simulink model "component_contoller_PID"  (R2025a)
settings: Solver=FixedStepAuto  StartTime=0.0  StopTime=10.0  RelTol=1e-3  EnableMultiTasking=on
undefined symbols (not defined in the file): break_pedal_percentage, gas_pedal_percentage, steering_wheel_angle
libraries: slpidlib x1, drivingvehiclecontroller x1
settings Model: Creator=chmurski  LastModifiedBy=MarikL
settings SolverCC: AlgebraicLoopSolver=TrustRegion  PositivePriorityOrder=on
settings OptimizationCC: EnhancedBackFolding=on  PassReuseOutputArgsAs=Individual arguments  ZeroExternalMemoryAtStartup=off  ZeroInternalMemoryAtStartup=off  MaxStackSize=2048  OptimizeBlockOrder=speed  DifferentSizesBufferReuse=on  OptimizationCustomize=off  EfficientTunableParamExpr=on
settings DebuggingCC: ParameterTunabilityLossMsg=error  UnconnectedInputMsg=warning  UnconnectedOutputMsg=warning  UnconnectedLineMsg=warning
settings HardwareCC: ProdBitPerPointer=32.0  ProdBitPerSizeT=32.0  ProdBitPerPtrDiffT=32.0  ProdLargestAtomicInteger=Long  ProdWordSize=32.0  ProdLongLongMode=on  ProdHWDeviceType=Infineon->TriCore
settings ModelReferenceCC: EnableRefExpFcnMdlSchedulingChecks=on  ModelReferenceNumInstancesAllowed=Single
settings SFSimCC: MATLABDynamicMemAlloc=off
settings RTWCC: SystemTargetFile=ert.tlc  HardwareBoard=Infineon AURIX TC4x - TriBoards  TemplateMakefile=ert_default_tmf  Toolchain=TASKING SmartCode for TriCore  GPUComputeCapability=3.5  DLArmComputeVersion=19.05  Description=Embedded Coder
settings CodeAppCC: ForceParamTrailComments=on  IgnoreCustomStorageClasses=off  MaxIdLength=256.0  OperatorAnnotations=on  SimulinkDataObjDesc=on  SFDataObjDesc=on  InsertBlockDesc=on
settings ERTTargetCC: ExtModeTransport=0.0  ExtModeStaticAlloc=off  ExtModeMexFile=ext_comm  ExtModeIntrfLevel=Level1  InlinedParameterPlacement=Hierarchical  DynamicArrayContainerType=coder::array  SubcomponentCodeInterfacePackaging=Nonreusable function
settings SimscapeCC: SimscapeLogDataHistory=5000  SimscapeLogDecimation=1

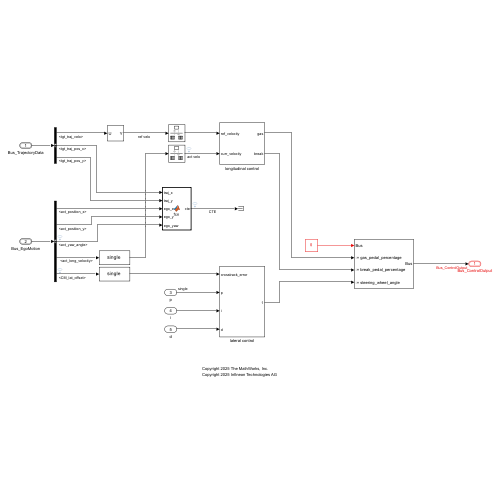
[thumbnail: Simulink's stored preview of the top-level diagram]
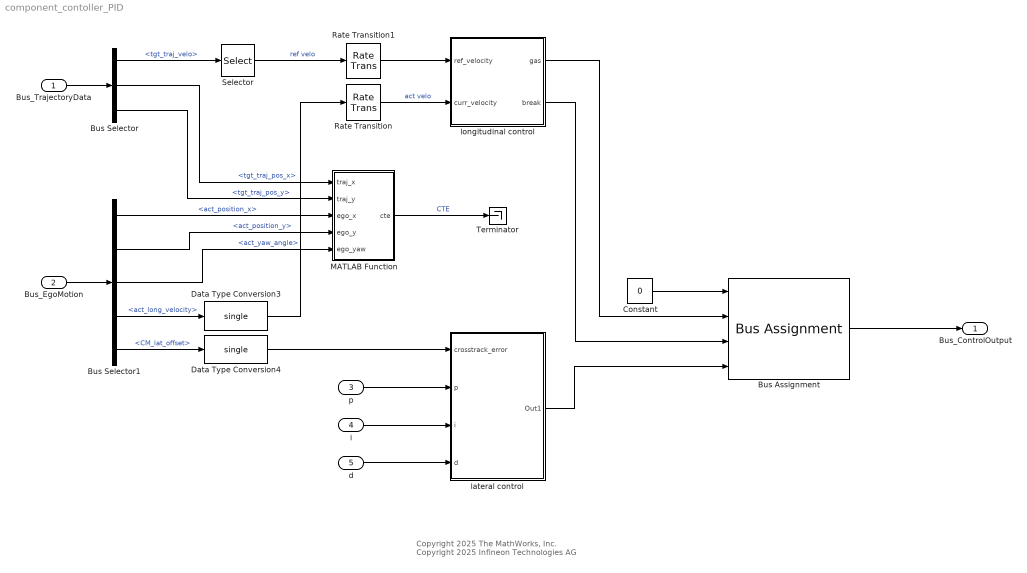
== system component_contoller_PID ==
  note: Copyright 2025 The MathWorks, Inc.
      | Copyright 2025 Infineon Technologies AG
  Bus_TrajectoryData : Inport  OutDataTypeStr=Bus: Bus_TrajectoryData
  Bus_EgoMotion : Inport  Port=2  OutDataTypeStr=Bus: Bus_EgoMotion
  p : Inport  Port=3  OutDataTypeStr=single
  i : Inport  Port=4
  d : Inport  Port=5
  Bus Assignment : BusAssignment  AssignedSignals=gas_pedal_percentage,break_pedal_percentage,steering_wheel_angle
  Bus Selector : BusSelector  OutputSignals=tgt_traj_velo,tgt_traj_pos_x,tgt_traj_pos_y
  Bus Selector1 : BusSelector  OutputSignals=act_position_x,act_position_y,act_yaw_angle,act_long_velocity,CM_lat_offset
  Constant : Constant  Value=0  OutDataTypeStr=Bus: Bus_ControlOutput  SampleTime=0.01
  Data Type Conversion3 : DataTypeConversion  OutDataTypeStr=single  SaturateOnIntegerOverflow=off  RndMeth=Floor
  Data Type Conversion4 : DataTypeConversion  OutDataTypeStr=single  SaturateOnIntegerOverflow=off  RndMeth=Floor
  MATLAB Function : MATLAB Function  TreatAsAtomicUnit=on
  Rate Transition : RateTransition
  Rate Transition1 : RateTransition
  Selector : Selector  InputPortWidth=50  IndexOptions=Index vector (dialog)  Indices=[1]  OutputSizes=1
  Terminator : Terminator
  lateral control : Subsystem
  longitudinal control : Subsystem
  Bus_ControlOutput : Outport  OutDataTypeStr=Bus: Bus_ControlOutput  VectorParamsAs1DForOutWhenUnconnected=off  BusOutputAsStruct=on
  wires:
  Rate Transition/1 -> longitudinal control/2(curr_velocity)  "act velo"
  Rate Transition1/1 -> longitudinal control/1(ref_velocity)
  d/1 -> lateral control/4(d)
  Bus Selector1/5 -> Data Type Conversion4/1  "<CM_lat_offset>"
  Constant/1 -> Bus Assignment/1
  Bus Selector1/4 -> Data Type Conversion3/1  "<act_long_velocity>"
  Selector/1 -> Rate Transition1/1  "ref velo"
  i/1 -> lateral control/3(i)
  Bus Assignment/1 -> Bus_ControlOutput/1
  p/1 -> lateral control/2(p)
  Bus_TrajectoryData/1 -> Bus Selector/1
  lateral control/1(Out1) -> Bus Assignment/4
  longitudinal control/2(break) -> Bus Assignment/3
  longitudinal control/1(gas) -> Bus Assignment/2
  Bus Selector/1 -> Selector/1  "<tgt_traj_velo>"
  Bus Selector/2 -> MATLAB Function/1(traj_x)  "<tgt_traj_pos_x>"
  Bus Selector/3 -> MATLAB Function/2(traj_y)  "<tgt_traj_pos_y>"
  Bus_EgoMotion/1 -> Bus Selector1/1
  MATLAB Function/1(cte) -> Terminator/1  "CTE"
  Bus Selector1/1 -> MATLAB Function/3(ego_x)  "<act_position_x>"
  Bus Selector1/2 -> MATLAB Function/4(ego_y)  "<act_position_y>"
  Bus Selector1/3 -> MATLAB Function/5(ego_yaw)  "<act_yaw_angle>"
  Data Type Conversion3/1 -> Rate Transition/1
  Data Type Conversion4/1 -> lateral control/1(crosstrack_error)

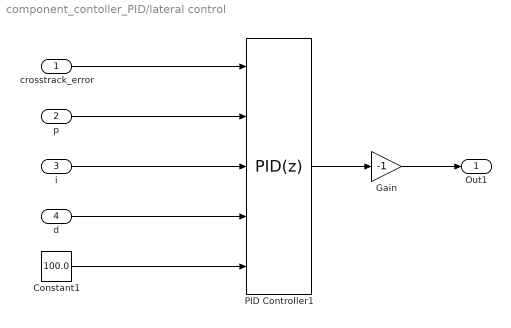
== system component_contoller_PID/lateral control ==
  crosstrack_error : Inport
  p : Inport  Port=2
  i : Inport  Port=3
  d : Inport  Port=4
  Constant1 : Constant  Value=100.0  OutDataTypeStr=single
  Gain : Gain  Gain=-1
  PID Controller1 : slpidlib/PID Controller  Controller=PID  Form=Parallel  TimeDomain=Discrete-time  UseExternalTs=off  SampleTime=0.01  IntegratorMethod=Forward Euler  FilterMethod=Forward Euler  ControllerParametersSource=external  P=1  I=1  UseKiTs=off  D=0  UseExternalDerivativeSource=off  N=100  UseFilter=on  TunerSelectOption=Transfer Function Based (PID Tuner App)  InitialConditionSource=internal  InitialConditionForIntegrator=0  InitialConditionForFilter=0  DifferentiatorICPrevScaledInput=0  ExternalReset=none  TrackingMode=off  Kt=1  LimitOutput=off  SatLimitsSource=internal  UpperSaturationLimit=1  LowerSaturationLimit=-1  LinearizeAsGain=on  AntiWindupMode=none  Kb=1  LimitIntegrator=off  UpperIntegratorSaturationLimit=inf  LowerIntegratorSaturationLimit=-inf  POutMin=[]  POutMax=[]  IOutMin=[]  IOutMax=[]  DOutMin=[]  DOutMax=[]  NOutMin=[]  NOutMax=[]  SumOutMin=[]  SumOutMax=[]  SaturationOutMin=[]  SaturationOutMax=[]  PParamMin=[]  PParamMax=[]  IParamMin=[]  IParamMax=[]  DParamMin=[]  DParamMax=[]  NParamMin=[]  NParamMax=[]  KbParamMin=[]  KbParamMax=[]  KtParamMin=[]  KtParamMax=[]  KbOutMin=[]  KbOutMax=[]  KtOutMin=[]  KtOutMax=[]  IntegratorOutMin=[]  IntegratorOutMax=[]  FilterOutMin=[]  FilterOutMax=[]  SumI1OutMin=[]  SumI1OutMax=[]  SumI2OutMin=[]  SumI2OutMax=[]  SumI3OutMin=[]  SumI3OutMax=[]  SumI4OutMin=[]  SumI4OutMax=[]  SumDOutMin=[]  SumDOutMax=[]  DifferentiatorOutMin=[]  DifferentiatorOutMax=[]  FilterDiffOutCoefMin=[]  FilterDiffOutCoefMax=[]  ReciprocalOutMin=[]  ReciprocalOutMax=[]  SumDenOutMin=[]  SumDenOutMax=[]  SumNumOutMin=[]  SumNumOutMax=[]  DivideOutMin=[]  DivideOutMax=[]  UdiffTsProdOutMin=[]  UdiffTsProdOutMax=[]  NTsProdOutMin=[]  NTsProdOutMax=[]  UintegralTsProdOutMin=[]  UintegralTsProdOutMax=[]  UngainTsProdOutMin=[]  UngainTsProdOutMax=[]  ClampingZeroOutDataTypeStr=Inherit: Inherit via back propagation  ClampingZeroOutMin=[]  ClampingZeroOutMax=[]  FilterDenConstantOutDataTypeStr=Inherit: Inherit via back propagation  FilterDenConstantOutMin=[]  FilterDenConstantOutMax=[]  PCopyOutDataTypeStr=Inherit: Inherit via back propagation  PCopyOutMin=[]  PCopyOutMax=[]  NCopyOutDataTypeStr=Inherit: Inherit via back propagation  NCopyOutMin=[]  NCopyOutMax=[]  IntegratorContinuousStateAttributes=''  IntegratorStateMustResolveToSignalObject=off  IntegratorRTWStateStorageClass=Auto  FilterContinuousStateAttributes=''  FilterStateMustResolveToSignalObject=off  FilterRTWStateStorageClass=Auto  ParallelPVariant=ExternalParameters  IdealPVariant=Disabled  IVariant=ExternalParameters  DVariant=ExternalParameters  IntegratorVariant=Discrete  SatVariant=Disabled  AWVariant=Passthrough  PCopyVariant=Disabled  TRVariant=Disabled  FdbkBlocksVariant=Forward  IdealPFdbkVariant=Disabled  SatFdbkVariant=Disabled  DerivativeFilterVariant=ForwardEulerFilter  NVariant=ExternalParameters  NCopyVariant=Disabled  FilterICVariant=InternalICsFilter  IntegratorICVariant=InternalICs  ExternalResetVariant=Disabled  TRSumVariant=Passthrough  SumFdbkVariant=Disabled  SumVariant=Sum_PID  TsampFilterVariant=InternalTs  TsampNgainVariant=Passthrough  TsampIntegralVariant=Disabled_SignalSpec  ExternalSaturationOutDataTypeStr=Inherit: Same as second input  DerivativeSourceVariant=ErrorSignal  PreIntVariant=InternalPreInt
  Out1 : Outport
  wires:
  PID Controller1/1 -> Gain/1
  Constant1/1 -> PID Controller1/5
  Gain/1 -> Out1/1
  crosstrack_error/1 -> PID Controller1/1
  p/1 -> PID Controller1/2
  i/1 -> PID Controller1/3
  d/1 -> PID Controller1/4

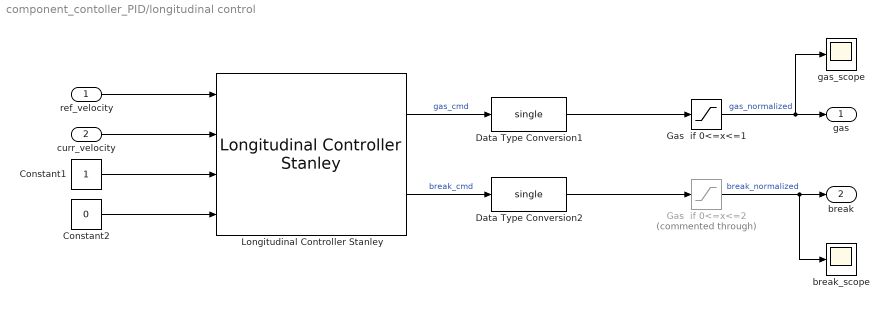
== system component_contoller_PID/longitudinal control ==
  ref_velocity : Inport
  curr_velocity : Inport  Port=2
  Constant1 : Constant  OutDataTypeStr=single
  Constant2 : Constant  Value=0  OutDataTypeStr=single
  Data Type Conversion1 : DataTypeConversion  OutDataTypeStr=single  SaturateOnIntegerOverflow=off  RndMeth=Floor
  Data Type Conversion2 : DataTypeConversion  OutDataTypeStr=single  SaturateOnIntegerOverflow=off  RndMeth=Floor
  Gas  if 0<=x<=1 : Saturate  UpperLimit=1  LowerLimit=0
  Gas  if 0<=x<=2 : Saturate  Commented=through  UpperLimit=1  LowerLimit=0
  Longitudinal Controller Stanley : drivingvehiclecontroller/Longitudinal Controller Stanley  Kp=0.35  Ki=2.5  SampleTime=0.01  MaxAcceleration=3  MaxDeceleration=6
  break_scope : Scope
      settings: ActiveDisplayYMinimum=-1  ActiveDisplayYMaximum=1  DataLoggingVariableName=ScopeData3
  gas_scope : Scope
      settings: ActiveDisplayYMinimum=0.9  ActiveDisplayYMaximum=1.1  DataLoggingVariableName=ScopeData2
  gas : Outport
  break : Outport  Port=2
  wires:
  Gas  if 0<=x<=1/1 -> gas/1, gas_scope/1  "gas_normalized"
  Constant1/1 -> Longitudinal Controller Stanley/3
  Constant2/1 -> Longitudinal Controller Stanley/4
  Longitudinal Controller Stanley/1 -> Data Type Conversion1/1  "gas_cmd"
  Longitudinal Controller Stanley/2 -> Data Type Conversion2/1  "break_cmd"
  curr_velocity/1 -> Longitudinal Controller Stanley/2
  ref_velocity/1 -> Longitudinal Controller Stanley/1
  Gas  if 0<=x<=2/1 -> break_scope/1, break/1  "break_normalized"
  Data Type Conversion1/1 -> Gas  if 0<=x<=1/1
  Data Type Conversion2/1 -> Gas  if 0<=x<=2/1

== matlab function component_contoller_PID/MATLAB Function ==
  data: traj_x input; cte output; traj_y input; ego_x input; ego_y input; ego_yaw input
function cte = fcn(traj_x, traj_y, ego_x, ego_y, ego_yaw)

cte = calculate_cross_track_error(traj_x, traj_y, ego_x, ego_y, ego_yaw);
